simulink model "speed_m_per_s_to_km_per_hr"  (R2020b)
settings: Solver=VariableStepAuto  StartTime=0.0  StopTime=10.0  RelTol=1e-3
settings Model: Creator=Training  LastModifiedBy=Training

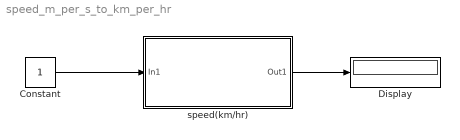
== system speed_m_per_s_to_km_per_hr ==
  Constant : Constant
  Display : Display
  speed(km/hr) : Subsystem
  wires:
  speed(km/hr)/1(Out1) -> Display/1
  Constant/1 -> speed(km/hr)/1(In1)

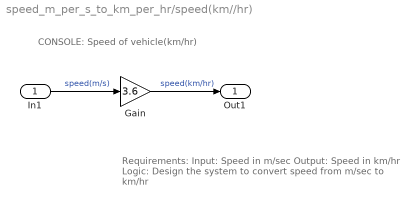
== system speed_m_per_s_to_km_per_hr/speed(km//hr) ==
  note: CONSOLE: Speed of vehicle(km/hr)
  note: Requirements:
      | Input: Speed in m/sec
      | Output: Speed in km/hr
      | Logic: Design the system to convert speed from m/sec to km/hr
  In1 : Inport
  Gain : Gain  Gain=3.6
  Out1 : Outport
  wires:
  In1/1 -> Gain/1  "speed(m/s)"
  Gain/1 -> Out1/1  "speed(km/hr)"
